simulink model "controller_test_lqe_2"  (R2015a)
settings: Solver=FixedStepDiscrete  StartTime=0.0  StopTime=40  FixedStep=0.02  RelTol=1e-3
undefined symbols (not defined in the file or in its folder): A, B, C, CE, DE, GAMMAE, PHIE
settings Model: ExtModeTrigDuration=200000  Creator=alunos  LastModifiedBy=jmgri
settings DataIOCC: LimitDataPoints=off
settings HardwareCC: ProdBitPerPointer=64  ProdLargestAtomicFloat=Float  ProdIntDivRoundTo=Zero  ProdEndianess=LittleEndian  ProdHWDeviceType=Specified  TargetIntDivRoundTo=Zero  TargetEndianess=LittleEndian  TargetHWDeviceType=Intel->x86/Pentium
settings RTWCC: SystemTargetFile=rtwin.tlc  TemplateMakefile=rtwin.tmf  Description=Simulink Desktop Real-Time  RTWCompilerOptimization=on
settings CodeAppCC: MaxIdLength=95
settings RTWinTargetCC: TargetPreCompLibLocation=C:\Program Files\MATLAB\R2017a\toolbox\sldrt\lib\win64  GeneratePreprocessorConditionals=Use local settings  ExtModeMexFile=sldrtext

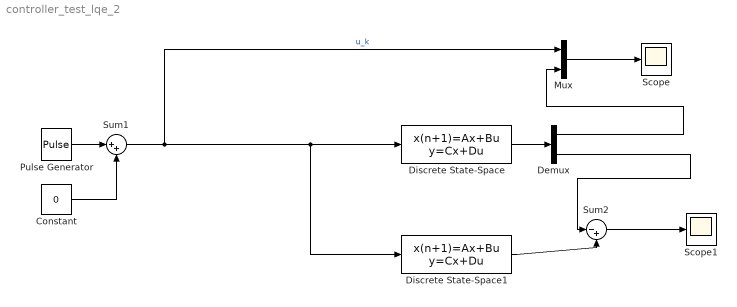
== system controller_test_lqe_2 ==
  Constant : Constant  Value=0
  Demux : Demux  Outputs=[1 length(A)]
  Discrete State-Space : DiscreteStateSpace  A=A  B=B  C=[C;eye(length(A))]  D=[0;zeros(length(A),1)]  SampleTime=-1
  Discrete State-Space1 : DiscreteStateSpace  A=PHIE  B=GAMMAE  C=CE  D=DE  SampleTime=-1
  Mux : Mux  Inputs=2
  Pulse Generator : DiscretePulseGenerator  PulseType=Time based  Period=3  PulseWidth=50
  Scope : Scope
      settings: TickLabels=on  SaveName=simulation_data  SampleInput=on
  Scope1 : Scope
      settings: TickLabels=on  SaveName=simulation_data1  SampleInput=on
  Sum1 : Sum  Inputs=|++
  Sum2 : Sum  Inputs=|-+
  wires:
  Sum1/1 -> Mux/1, Discrete State-Space1/1, Discrete State-Space/1  "u_k"
  Mux/1 -> Scope/1
  Demux/1 -> Mux/2
  Discrete State-Space/1 -> Demux/1
  Pulse Generator/1 -> Sum1/1
  Constant/1 -> Sum1/2
  Demux/2 -> Sum2/1
  Discrete State-Space1/1 -> Sum2/2
  Sum2/1 -> Scope1/1
